simulink model "Demo1"  (Simulink 6.5)
settings: Solver=FixedStepDiscrete  SolverMode=SingleTasking  StartTime=0.0  StopTime=1.5  FixedStep=Ts  RelTol=1e-3
InitFcn:
  | Ts=2e-6;  load power_svpwm_init;
undefined symbols (not defined in the file): DiscIntNeverNeededParam, powergui, x
libraries: powerlib x10, powerlib_extras x9
settings Model: Creator=Gilber Sybille, IREQ  LastModifiedBy=RS  ExtModeAutoUpdateStatusClock=off
settings DataIOCC: LimitDataPoints=off  LoadInitialState=on  SaveFinalState=on  SaveOutput=off  SaveTime=off  SignalLoggingName=sigsOut
settings OptimizationCC: BooleanDataType=off  InlineInvariantSignals=on
settings DebuggingCC: CheckExecutionContextPreStartOutputMsg=on  CheckExecutionContextRuntimeOutputMsg=on  SolverPrmCheckMsg=none  MultiTaskDSMMsg=warning  MultiTaskCondExecSysMsg=none  StrictBusMsg=None
settings HardwareCC: TargetUnknown=on
settings RTWCC: IncludeERTFirstTime=on

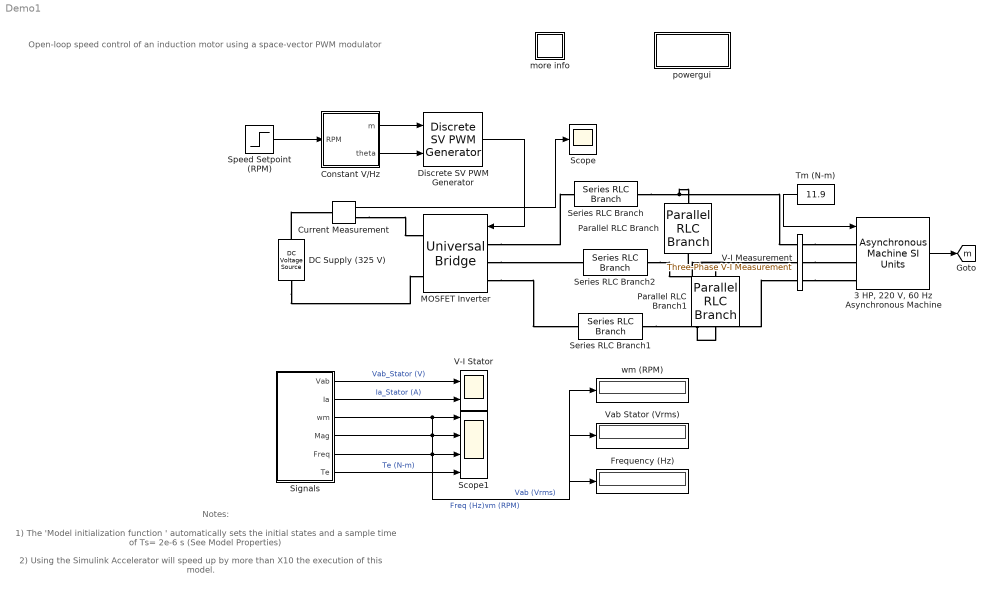
== system Demo1 ==
  note: Open-loop speed control of an induction motor using
      | a space-vector PWM modulator
  note: 1) The 'Model initialization function ' automatically sets  the initial states
      |     and a sample time of Ts= 2e-6 s  (See Model Properties)
  note: 2) Using the Simulink Accelerator will speed up by more
      |      than X10 the execution of this model.
  note: Notes:
  "3 HP, 220 V, 60 Hz Asynchronous Machine" : powerlib/Machines/Asynchronous Machine SI Units  DialogController=PMDialogs.PMDefaultMaskDlg  SystemSampleTime=-1  PresetModel=No  MechanicalLoad=Torque Tm  ShowDetailedParameters=on  RotorType=Squirrel-cage  ReferenceFrame=Stationary  NominalParameters=[ 3*746, 220, 60 ]  Stator="[ 0.435  2*2.0e-3 ]"  Rotor="[ 0.816  2.0e-3 ]"  Lm=69.31e-3  Mechanical="[ 0.089  0  2 ]"  PolePairs=2  Units=1  LoadFlowParameters=2000  SimulateSaturation=off  Saturation=[0 0;0 0]
  Constant V/Hz : Subsystem
  Current Measurement : powerlib/Measurements/Current Measurement  DialogController=PMDialogs.PMDefaultMaskDlg  SystemSampleTime=-1  PhasorSimulation=off  OutputType=Complex  PSBequivalent=0
  DC Supply (325 V) : powerlib/Electrical Sources/DC Voltage Source  Orientation=up  DialogController=PMDialogs.PMDefaultMaskDlg  SystemSampleTime=-1  Amplitude=325  Measurements=None
  Discrete SV PWM Generator : powerlib_extras/Discrete  Control Blocks/Discrete SV PWM Generator  DialogController=PMDialogs.PMDefaultMaskDlg  SystemSampleTime=-1  InputType=Magnitude-Angle (rad)  SwitchingPattern=Pattern #1  Fc=1980  ParUref=[0.8 -30 50]  Ts=Ts
  Frequency (Hz) : Display
      settings: Format=bank  SampleTime=Ts*1000
  MOSFET Inverter : powerlib/Power Electronics/Universal Bridge  Orientation=left  DialogController=PMDialogs.PMDefaultMaskDlg  SystemSampleTime=-1  Arms=3  SnubberResistance=1e5  SnubberCapacitance=inf  Device=MOSFET / Diodes  Ron=0.2e-3  Lon=0  ForwardVoltages="[  0  0  ]"  ForwardVoltage=0  GTOparameters=[ 10e-6 , 20e-6 ]  IGBTparameters=[ 1e-6 , 2e-6 ]  Measurements=None  converterType=Rectifier
  Parallel RLC Branch : powerlib/Elements/Parallel RLC Branch  Orientation=down  DialogController=PMDialogs.PMDefaultMaskDlg  PhysicalDomain=powersysdomain  SubClassName=unknown  LeftPortType=p1  RightPortType=p1  LConnTagsString=a  RConnTagsString=__new0  BranchType=RLC  Resistance=100000  Inductance=80e-3  SetiL0=off  InitialCurrent=0  Capacitance=127e-6  Setx0=off  InitialVoltage=0  Measurements=None
  Parallel RLC Branch1 : powerlib/Elements/Parallel RLC Branch  Orientation=down  DialogController=PMDialogs.PMDefaultMaskDlg  PhysicalDomain=powersysdomain  SubClassName=unknown  LeftPortType=p1  RightPortType=p1  LConnTagsString=a  RConnTagsString=__new0  BranchType=RLC  Resistance=100000  Inductance=80e-3  SetiL0=off  InitialCurrent=0  Capacitance=127e-6  Setx0=off  InitialVoltage=0  Measurements=None
  Scope : Scope
      settings: MaxDataPoints=10000000  SampleInput=on  SampleTime=10e-6
  Scope1 : Scope  NumInputPorts=4
      settings: TimeRange=1.5  YMin=1200~160~40~5  YMax=1800~240~70~15  SaveName=VI_Stator1  SampleInput=on  SampleTime=Ts*100
  Series RLC Branch : powerlib/Elements/Series RLC Branch  DialogController=PMDialogs.PMDefaultMaskDlg  PhysicalDomain=powersysdomain  SubClassName=unknown  LeftPortType=p1  RightPortType=p1  LConnTagsString=__new0  RConnTagsString=__new0  BranchType=RLC  Resistance=1  Inductance=40e-3  SetiL0=off  InitialCurrent=0  Capacitance=256e-6  Setx0=off  InitialVoltage=0  Measurements=None
  Series RLC Branch1 : powerlib/Elements/Series RLC Branch  DialogController=PMDialogs.PMDefaultMaskDlg  PhysicalDomain=powersysdomain  SubClassName=unknown  LeftPortType=p1  RightPortType=p1  LConnTagsString=__new0  RConnTagsString=__new0  BranchType=RLC  Resistance=1  Inductance=40e-3  SetiL0=off  InitialCurrent=0  Capacitance=256e-6  Setx0=off  InitialVoltage=0  Measurements=None
  Series RLC Branch2 : powerlib/Elements/Series RLC Branch  DialogController=PMDialogs.PMDefaultMaskDlg  PhysicalDomain=powersysdomain  SubClassName=unknown  LeftPortType=p1  RightPortType=p1  LConnTagsString=__new0  RConnTagsString=__new0  BranchType=RLC  Resistance=1  Inductance=40e-3  SetiL0=off  InitialCurrent=0  Capacitance=256e-6  Setx0=off  InitialVoltage=0  Measurements=None
  Signals : Subsystem
  Speed Setpoint (RPM) : Step  Time=0.05  After=1500  SampleTime=Ts
  Tm (N-m) : Constant  Orientation=left  Value=11.9  OutDataType=sfix(16)  ConRadixGroup=Use specified scaling  OutScaling=2^0  SampleTime=inf  FramePeriod=inf
  V-I Measurement : powerlib/Measurements/Three-Phase V-I Measurement  DialogController=PMDialogs.PMDefaultMaskDlg  SystemSampleTime=-1  VoltageMeasurement=phase-to-phase  SetLabelV=on  LabelV=Vabc_Stator  Vpu=off  CurrentMeasurement=yes  SetLabelI=on  LabelI=Iabc_Stator  Ipu=off  Pbase=100e6  Vbase=500e3  OutputType=Magnitude  PhasorSimulation=off  PSBequivalent=0
  V-I Stator : Scope  NumInputPorts=2
      settings: TimeRange=0.1  YMin=-400~-25  YMax=400~25  SaveName=VI_Stator  SampleInput=on  SampleTime=Ts*5
  Vab Stator (Vrms) : Display
      settings: Format=bank  SampleTime=Ts*1000
  more info : Subsystem
      settings: OpenFcn=showdemo(bdroot(gcb))
      mask Display: disp('?')
  powergui : Subsystem  Priority=2  AncestorBlock=powerlib/powergui  InitFcn=powergui( 'InitFcn_Callback' , gcb , 0 , [ ] );  mask(PSB option menu block){SimulationMode=Discrete, SampleTime=Ts, echomessages=off, RestoreLinks=warning, x0status=blocks, Frange=[0:2:500], Ylog=off, Xlog=on, ShowGrid=off, save=off, variable=ZData, structure=VI_Stator, ZoomFFT=on, StartTime=0.05, cycles=2, DisplayStyle=1, fundamental=60, FreqAxis=off, MaxFrequency=5000, frequencyindice=60, frequencyindicesteady=1, RmsSteady=1, display=off, Ts=0, frequency=60, methode=off, HookPort=off, Interpol=off}
      mask prompts: SimulationMode "Simulation mode"; SampleTime "Sample time Ts (when simulation mode is Discrete) (s)"; echomessages "Echo  Messages"; RestoreLinks "Restore disabled links"; x0status "Initial electrical states status"; Frange "Impedance tool: Frequency Range"; Ylog "Impedance tool: Log impedance"; Xlog "Impedance tool: log Frequency"; ShowGrid "Impedance tool: grid"; save "Impedance tool: Save Data To Workspace"; variable "Impedance tool: Variable Name"; structure "Structure Name (PSBFFTSCOPE)"; ZoomFFT "ZoomFFT (PSBFFTSCOPE)"; StartTime "Start Time (PSBFFTSCOPE)"; cycles "Cycles (PSBFFTSCOPE)"; DisplayStyle "Display style (PSBFFTSCOPE)"; fundamental "Fundamental (PSBFFTSCOPE)"; FreqAxis "Frequency Axis (PSBFFTSCOPE)"; MaxFrequency "Max Frequency (PSBFFTSCOPE)"; frequencyindice "Load flow frequency (Hz)"; frequencyindicesteady "Frequency indice (STEADYSTATE)"; RmsSteady "RMS display (STEADYSTATE)"; display "Display Results"; Ts "OBSOLETE 1"; frequency "Phasor frequency (Hz)"; methode "Phasor simulation"; HookPort "Hook port"; Interpol "Interpolate"
      mask init:
      | powerlibroot = which('powersysdomain');
      | PSBroot = powerlibroot(1:end-16);
      | %
      | switch SimulationMode
      | 	case 1
      | 		message=sprintf('Continuous');
      | 	case 2
      |         SampleTimeeval=evalin('base',SampleTime,'NaN');
      |         if isnan(SampleTimeeval)
      |             message=sprintf('Warning !!,\nUndefined sample time');
      |         else
      |             message=sprintf('Discrete,\nTs = %.4g s.',SampleTimeeval);
      |         end
      | 	case 3
      | 		message=sprintf('Phasors');
      | end
      | if strcmp(bdroot,'powerlib')
      |   message='powergui';
      | end
      | power_initmask();
      settings: CopyFcn=powergui( 'Copy_Callback' , gcb , 0 , [ ] );  ModelCloseFcn=powergui( 'CloseButton_Callback' , gcb , [ ] , [ ] );  PreSaveFcn=powergui( 'CloseButton_Callback' , gcb , [ ] , [ ] );  NameChangeFcn=powergui( 'NameChangeFcn_Callback' , gcb , 0 , [ ] );
      settings: DeleteFcn=|
      | powergui( 'Copy_Callback' , gcb , 1 , [ ] );
      | powergui( 'CloseButton_Callback' , gcb , [ ] , [ ] );
      settings: OpenFcn=|
      | if (power_openblockproxy ('secondary'))
      | powergui(gcb,'PM')
      | end;
      mask Help: web(psbhelp)
      mask StyleString: popup(Continuous|Discrete|Phasor),edit,checkbox,popup(yes|warning|no),popup(blocks|steady|zero),edit,checkbox,checkbox,checkbox,checkbox,edit,edit,checkbox,edit,edit,edit,edit,checkbox,edit,edit,edit,edit,checkbox,edit,edit,checkbox,checkbox,checkbox
      mask CallbackString: ||||||||||||||||||||||||||powergui('HookPort',[],[],gcb);|
      mask Display: disp(message)
  wm (RPM) : Display
      settings: SampleTime=Ts*1000
  tag scope: m=global
  wires:
  "3 HP, 220 V, 60 Hz Asynchronous Machine"/1 -> [m]
  Constant V/Hz/2(theta) -> Discrete SV PWM Generator/2
  Signals/1(Vab) -> V-I Stator/1  "Vab_Stator (V)"
  Signals/2(Ia) -> V-I Stator/2  "Ia_Stator (A)"
  Signals/6(Te) -> Scope1/4  "Te (N-m)"
  Constant V/Hz/1(m) -> Discrete SV PWM Generator/1
  Discrete SV PWM Generator/1 -> MOSFET Inverter/1
  Signals/3(wm) -> Scope1/1, wm (RPM)/1  "wm (RPM)"
  Signals/4(Mag) -> Scope1/2, Vab Stator (Vrms)/1  "Vab (Vrms)"
  Signals/5(Freq) -> Scope1/3, Frequency (Hz)/1  "Freq (Hz)"
  Speed Setpoint (RPM)/1 -> Constant V/Hz/1(RPM)
  Current Measurement/1 -> Scope/1
  Tm (N-m)/1 -> "3 HP, 220 V, 60 Hz Asynchronous Machine"/1
  connections:
  DC Supply (325 V)/LConn1 -- MOSFET Inverter/RConn2
  V-I Measurement/RConn1 -- "3 HP, 220 V, 60 Hz Asynchronous Machine"/LConn1
  V-I Measurement/RConn2 -- "3 HP, 220 V, 60 Hz Asynchronous Machine"/LConn2
  V-I Measurement/RConn3 -- "3 HP, 220 V, 60 Hz Asynchronous Machine"/LConn3
  DC Supply (325 V)/RConn1 -- Current Measurement/LConn1
  Current Measurement/RConn1 -- MOSFET Inverter/RConn1
  MOSFET Inverter/LConn1 -- Series RLC Branch/LConn1
  Series RLC Branch/RConn1 -- V-I Measurement/LConn1 -- Parallel RLC Branch/LConn1
  MOSFET Inverter/LConn3 -- Series RLC Branch1/LConn1
  Series RLC Branch1/RConn1 -- V-I Measurement/LConn3 -- Parallel RLC Branch1/RConn1
  V-I Measurement/LConn2 -- Parallel RLC Branch1/LConn1 -- Parallel RLC Branch/RConn1 -- Series RLC Branch2/RConn1
  MOSFET Inverter/LConn2 -- Series RLC Branch2/LConn1

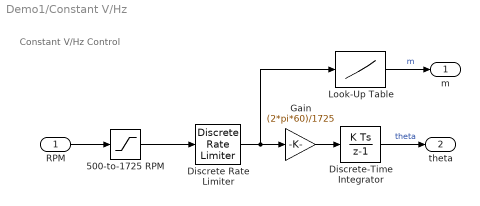
== system Demo1/Constant V/Hz ==
  note: Constant V/Hz
      | Control
  RPM : Inport
  500-to-1725 RPM : Saturate  UpperLimit=1725  LowerLimit=500
  Discrete Rate Limiter : powerlib_extras/Discrete  Control Blocks/Discrete Rate Limiter  DialogController=PMDialogs.PMDefaultMaskDlg  SystemSampleTime=-1  R=500  F=-500  Vinit=1725  Ts=Ts
  Discrete-Time Integrator : DiscreteIntegrator  SampleTime=Ts  ICPrevOutput=DiscIntNeverNeededParam  ICPrevScaledInput=DiscIntNeverNeededParam
  Gain : Gain  Gain=(2*pi*60)/1725  SaturateOnIntegerOverflow=on
  Look-Up Table : Lookup  InputValues=[500 1725 2500]  OutputValues=[0.29 1 1]*0.957  LookUpMeth=Interpolation-Extrapolation  OutDataType=sfix(16)  OutScaling=2^0  SaturateOnIntegerOverflow=on  SampleTime=-1  LUTDesignTableMode=Redesign Table  LUTDesignDataSource=Block Dialog  LUTDesignFunctionName=sqrt(x)  LUTDesignUseExistingBP=on  LUTDesignRelError=0.01  LUTDesignAbsError=1e-6  RndMeth=Floor
      settings: LockScale=off
  m : Outport
  theta : Outport  Port=2
  wires:
  Gain/1 -> Discrete-Time Integrator/1
  Discrete Rate Limiter/1 -> Gain/1, Look-Up Table/1
  Look-Up Table/1 -> m/1  "m"
  RPM/1 -> 500-to-1725 RPM/1
  Discrete-Time Integrator/1 -> theta/1  "theta"
  500-to-1725 RPM/1 -> Discrete Rate Limiter/1

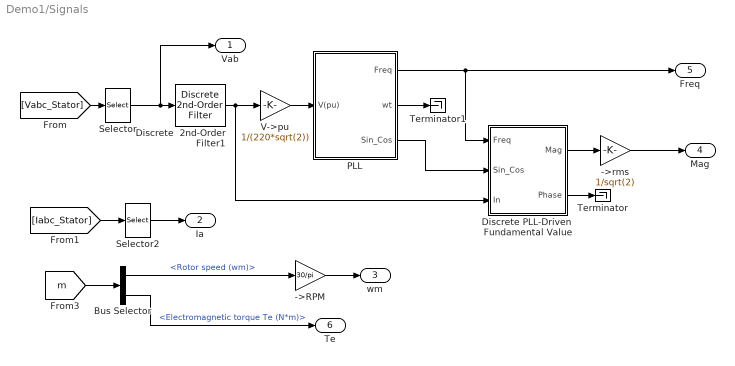
== system Demo1/Signals ==
  ->RPM : Gain  Gain=30/pi  SaturateOnIntegerOverflow=on
  ->rms : Gain  Gain=1/sqrt(2)  SaturateOnIntegerOverflow=on
  Bus Selector : BusSelector  OutputSignals=Mechanical.Rotor speed (wm),Mechanical.Electromagnetic torque Te (N*m)
  Discrete PLL-Driven  Fundamental Value : Subsystem  mask(Discrete PLL-Driven Fundamental Value){Finit=60, Par_Init=[220*sqrt(2) 0], Ts=Ts*20}
      mask prompts: Finit "Initial fundamental frequency (Hz):"; Par_Init "Initial input: [ Mag  Phase-relative-to-PLL(degrees) ]"; Ts "Sample time:"
      mask help:
      | This discrete block computes the fundamental value of the input signal (port In) over a running window of one cycle of a specified fundamental frequency (port Freq). Input port "Sin_Cos" (a two-dimension signal) provides the reference frame required for the computation..
      |  First and second outputs return respectively the magnitude and phase (in degrees relative to the PLL phase) of the fundamental.
      | For the first cycle of simulation, the ouputs are held constant to the values specified by the parameter "Initial input".
      mask init:
      | Real_Init=Par_Init(1)*cos(pi/180*Par_Init(2));
      | Imag_Init=Par_Init(1)*sin(pi/180*Par_Init(2));
  Discrete  2nd-Order Filter1 : powerlib_extras/Discrete  Control Blocks/Discrete  2nd-Order Filter  DialogController=PMDialogs.PMDefaultMaskDlg  SystemSampleTime=-1  FilterType=Lowpass  Fo=2000  Zeta=0.707  Ts=Ts  Initialize=on  Vac_Init=[1 30 60]  Vdc_Init=0  PlotResponse=off  param1=[1 500 1]
  PLL : Subsystem  mask(Discrete 1-phase PLL){Par_Init=[27.52 60], ParK=[120 2800], Ts=Ts*20}
      mask prompts: Par_Init "Initial input:[ Phase(degrees)   Frequency(Hz) ]"; ParK "Regulator gains [ Kp  Ki ]"; Ts "Sample time:"
      mask help:
      | This Phase Locked Loop (PLL) system can be used  to synchronize on a variable frequency sinusoidal signal.
      |
      | Input 1: Normalized input signal V(pu)
      |
      | Output 1:  Measured frequency (Hz) = w/(2pi)
      | Output 2:  Ramp w.t  varying between  0 and 2*pi, synchronized on the zero-crossing (rising) of  the input signal
      | Output 3: Vector [sin(wt) cos(wt)]
      mask init:
      | Kp=ParK(1);
      | Ki=ParK(2);
      | Phase_Init=Par_Init(1);
      | Finit=Par_Init(2);
  Selector : Selector  InputType=Vector  ElementSrc=Internal  Elements=[1]  RowSrc=Internal  Rows=1  ColumnSrc=Internal  Columns=1  InputPortWidth=3  IndexIsStartValue=off
  Selector2 : Selector  InputType=Vector  ElementSrc=Internal  Elements=[1]  RowSrc=Internal  Rows=1  ColumnSrc=Internal  Columns=1  InputPortWidth=3  IndexIsStartValue=off
  Terminator : Terminator
  Terminator1 : Terminator
  V->pu : Gain  Gain=1/(220*sqrt(2))  SaturateOnIntegerOverflow=on
  Vab : Outport
  Ia : Outport  Port=2
  wm : Outport  Port=3
  Mag : Outport  Port=4
  Freq : Outport  Port=5
  Te : Outport  Port=6
  wires:
  PLL/2(wt) -> Terminator1/1
  PLL/3(Sin_Cos) -> Discrete PLL-Driven  Fundamental Value/2(Sin_Cos)
  V->pu/1 -> PLL/1(V(pu))
  Selector/1 -> Vab/1, Discrete  2nd-Order Filter1/1
  Discrete PLL-Driven  Fundamental Value/1(Mag) -> ->rms/1
  [Vabc_Stator] -> Selector/1
  [Iabc_Stator] -> Selector2/1
  ->RPM/1 -> wm/1
  ->rms/1 -> Mag/1
  Selector2/1 -> Ia/1
  Discrete  2nd-Order Filter1/1 -> V->pu/1, Discrete PLL-Driven  Fundamental Value/3(In)
  [m] -> Bus Selector/1
  Bus Selector/1 -> ->RPM/1  "<Rotor speed (wm)>"
  Bus Selector/2 -> Te/1  "<Electromagnetic torque Te (N*m)>"
  PLL/1(Freq) -> Discrete PLL-Driven  Fundamental Value/1(Freq), Freq/1
  Discrete PLL-Driven  Fundamental Value/2(Phase) -> Terminator/1

== system Demo1/more info ==
  note: Pierre Giroux, Hydro-Quebec (IREQ)
  note: Start the simulation. Since the initial states values have been automatically loaded, the simulation should start in steady-state.
      | The initial motor speed should be 1720 RPM and the rms value of the stator voltages should be 220V@60Hz.
      |
      | At 0.1s, the speed setpoint is changed from 1725 to 1300 RPM.  You can observe the system dynamic looking inside
      | Scope 1. When the motor reaches a constant speed of 1275 RPM, the stator voltage rms value is down to 165.8V and
      | the frequency to 45.2 Hz.
      |
      | Stator voltage (phase AB) and phase A current waveforms can be observed in the "V-I Stator" Scope. You can do a FFT
      | of theses two quantities using the powergui FFT Analysis.
  note: Open-loop speed control of an induction motor using constant V/Hz principle and SV PWM technique
  note: Circuit Description
  note: Demonstration
  note: A 3-phase squirrel-cage motor rated 3 HP, 220 V, 60 Hz, 1725 rpm is fed by a 3-phase MOSFET inverter connected
      | to a DC voltage source of 325 V. The inverter is modeled using the "Universal Bridge" block and the motor by the
      | "Asynchronous Machine" block. Its stator leakage inductance Lls is set to twice its actual value to simulate the effect of a
      | smoothing reactor placed between the inverter  and the machine. The load torque applied to the  machine's shaft is
      | constant and set to its nominal value of 11.9 N.m.
      |
      | The firing pulses to the inverter are generated  by the "Space-Vector PWM modulator" block of the SPS library.
      | The chopping frequency is set to 1980 Hz and the input reference vector to "Magnitude-Angle".
      |
      | Speed control of the motor is performed by the "Constant V/Hz" block.  The magnitude and frequency of the stator voltages
      | are set based on the speed setpoint. By varying the stator voltages magnitude in proportion with frequency, the stator flux is
      | kept constant.

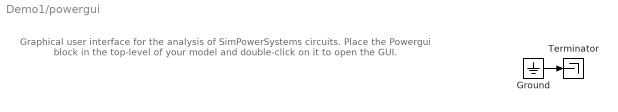
== system Demo1/powergui ==
  note: Graphical user interface for the analysis of  SimPowerSystems circuits.
      | Place the Powergui block in the top-level of your model and double-click
      | on it to open the GUI.
  Ground : Ground
  Terminator : Terminator
  wires:
  Ground/1 -> Terminator/1

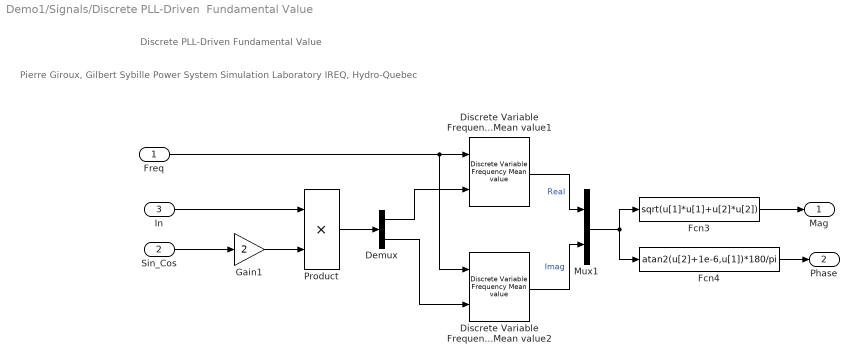
== system Demo1/Signals/Discrete PLL-Driven  Fundamental Value ==
  note: Discrete PLL-Driven Fundamental Value
  note: Pierre Giroux, Gilbert Sybille
      | Power System Simulation Laboratory
      | IREQ, Hydro-Quebec
  Freq : Inport
  Sin_Cos : Inport  Port=2
  In : Inport  Port=3
  Demux : Demux  Outputs=2
  Discrete Variable Frequency Mean value1 : powerlib_extras/Discrete Measurements/Discrete Variable Frequency Mean value  DialogController=PMDialogs.PMDefaultMaskDlg  SystemSampleTime=-1  Finit=Finit  Fmin=20  Vinit=Real_Init  Ts=Ts
  Discrete Variable Frequency Mean value2 : powerlib_extras/Discrete Measurements/Discrete Variable Frequency Mean value  DialogController=PMDialogs.PMDefaultMaskDlg  SystemSampleTime=-1  Finit=Finit  Fmin=20  Vinit=Imag_Init  Ts=Ts
  Fcn3 : Fcn  Expr=sqrt(u[1]*u[1]+u[2]*u[2])
  Fcn4 : Fcn  Expr=atan2(u[2]+1e-6,u[1])*180/pi
  Gain1 : Gain  Gain=2  SaturateOnIntegerOverflow=on
  Mux1 : Mux  Inputs=2
  Product : Product  SaturateOnIntegerOverflow=on  InputSameDT=on
  Mag : Outport
  Phase : Outport  Port=2
  wires:
  Mux1/1 -> Fcn3/1, Fcn4/1
  Fcn3/1 -> Mag/1
  Fcn4/1 -> Phase/1
  Discrete Variable Frequency Mean value2/1 -> Mux1/2  "Imag"
  Discrete Variable Frequency Mean value1/1 -> Mux1/1  "Real"
  Demux/1 -> Discrete Variable Frequency Mean value1/2
  Gain1/1 -> Product/2
  Product/1 -> Demux/1
  Demux/2 -> Discrete Variable Frequency Mean value2/2
  Freq/1 -> Discrete Variable Frequency Mean value2/1, Discrete Variable Frequency Mean value1/1
  Sin_Cos/1 -> Gain1/1
  In/1 -> Product/1

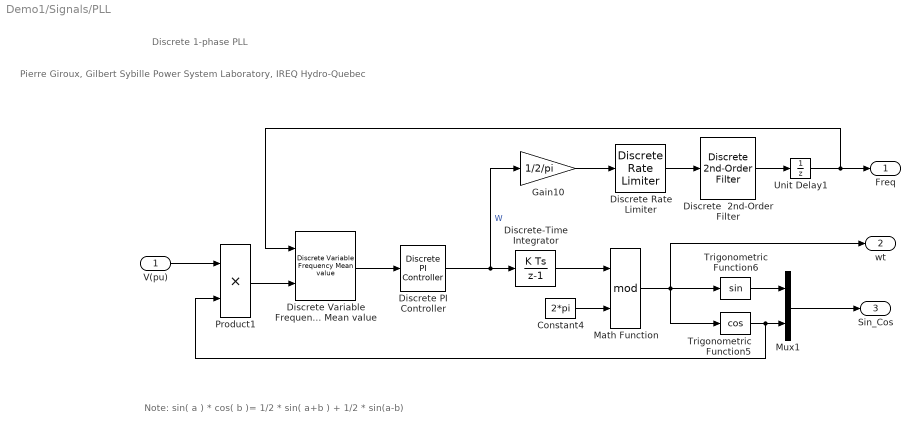
== system Demo1/Signals/PLL ==
  note: Pierre Giroux, Gilbert Sybille
      | Power System Laboratory, IREQ
      | Hydro-Quebec
  note: Note: sin( a ) * cos( b )= 1/2 * sin( a+b ) + 1/2 * sin(a-b)
  note: Discrete 1-phase PLL
  V(pu) : Inport
  Constant4 : Constant  Value=2*pi  OutDataType=sfix(16)  ConRadixGroup=Use specified scaling  OutScaling=2^0  SampleTime=inf  FramePeriod=inf
  Discrete PI Controller : powerlib_extras/Discrete  Control Blocks/Discrete PI Controller  DialogController=PMDialogs.PMDefaultMaskDlg  SystemSampleTime=-1  Kp=Kp  Ki=Ki  Par_Limits="[4  0.25]*2*pi*Finit"  Init=2*pi*Finit  Ts=Ts
  Discrete Rate Limiter : powerlib_extras/Discrete  Control Blocks/Discrete Rate Limiter  DialogController=PMDialogs.PMDefaultMaskDlg  SystemSampleTime=-1  R=30  F=-30  Vinit=Finit  Ts=Ts
  Discrete Variable Frequency Mean value : powerlib_extras/Discrete Measurements/Discrete Variable Frequency Mean value  DialogController=PMDialogs.PMDefaultMaskDlg  SystemSampleTime=-1  Finit=Finit  Fmin=10  Vinit=0  Ts=Ts
  Discrete  2nd-Order Filter : powerlib_extras/Discrete  Control Blocks/Discrete  2nd-Order Filter  DialogController=PMDialogs.PMDefaultMaskDlg  SystemSampleTime=-1  FilterType=Lowpass  Fo=25  Zeta=0.707  Ts=Ts  Initialize=on  Vac_Init="[0 0  Finit]"  Vdc_Init=Finit  PlotResponse=off  param1=[1 500 0.1]
  Discrete-Time Integrator : DiscreteIntegrator  InitialCondition=Phase_Init*pi/180  SampleTime=Ts  UpperSaturationLimit=0  LowerSaturationLimit=0  ICPrevOutput=DiscIntNeverNeededParam  ICPrevScaledInput=DiscIntNeverNeededParam
  Gain10 : Gain  Gain=1/2/pi  SaturateOnIntegerOverflow=on
  Math Function : Math  Operator=mod  SaturateOnIntegerOverflow=on
  Mux1 : Mux  Inputs=2
  Product1 : Product  SaturateOnIntegerOverflow=on  InputSameDT=on
  Trigonometric Function5 : Trigonometry  Operator=cos
  Trigonometric Function6 : Trigonometry
  Unit Delay1 : UnitDelay  X0=Finit  SampleTime=Ts
  Freq : Outport
  wt : Outport  Port=2
  Sin_Cos : Outport  Port=3
  wires:
  Unit Delay1/1 -> Discrete Variable Frequency Mean value/1, Freq/1
  Discrete PI Controller/1 -> Gain10/1, Discrete-Time Integrator/1  "W"
  V(pu)/1 -> Product1/1
  Constant4/1 -> Math Function/2
  Discrete-Time Integrator/1 -> Math Function/1
  Product1/1 -> Discrete Variable Frequency Mean value/2
  Discrete Variable Frequency Mean value/1 -> Discrete PI Controller/1
  Mux1/1 -> Sin_Cos/1
  Math Function/1 -> Trigonometric Function6/1, Trigonometric Function5/1, wt/1
  Trigonometric Function6/1 -> Mux1/1
  Trigonometric Function5/1 -> Mux1/2, Product1/2
  Discrete  2nd-Order Filter/1 -> Unit Delay1/1
  Gain10/1 -> Discrete Rate Limiter/1
  Discrete Rate Limiter/1 -> Discrete  2nd-Order Filter/1
